simulink model "fileSimulink"  (R2014a)
settings: Solver=ode45  StartTime=0.0  StopTime=3  RelTol=1e-3
libraries: cstblocks x2, simulink x2
settings Model: Creator=User  LastModifiedBy=User

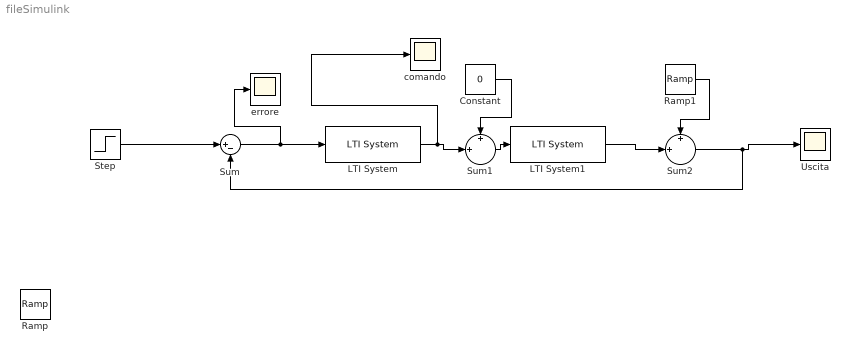
== system fileSimulink ==
  Constant : Constant  Value=0
  LTI System : cstblocks/LTI System  sys=Cz1  IC=[]
  LTI System1 : cstblocks/LTI System  sys=F  IC=[]
  Ramp : simulink/Sources/Ramp  slope=0  start=0  X0=0
  Ramp1 : simulink/Sources/Ramp  slope=0  start=0  X0=0
  Step : Step  Time=0  SampleTime=0
  Sum : Sum  Inputs=|+-
  Sum1 : Sum  Inputs=+|+||
  Sum2 : Sum  Inputs=+|+||
  "Uscita " : Scope
  "comando " : Scope
      settings: SaveName=ScopeData2
  "errore " : Scope
  wires:
  Sum/1 -> "errore "/1, LTI System/1
  Sum1/1 -> LTI System1/1
  LTI System/1 -> "comando "/1, Sum1/2
  Constant/1 -> Sum1/1
  Ramp1/1 -> Sum2/1
  LTI System1/1 -> Sum2/2
  Sum2/1 -> Sum/2, "Uscita "/1
  Step/1 -> Sum/1
